simulink model "p_regler_bei_u_max"  (R2016b)
settings: Solver=VariableStepAuto  StartTime=0.0  StopTime=10.0  RelTol=1e-3
undefined symbols (not defined in the file or in its folder): K_P
libraries: simulink x1
settings Model: Creator=Fritz  LastModifiedBy=Fritz

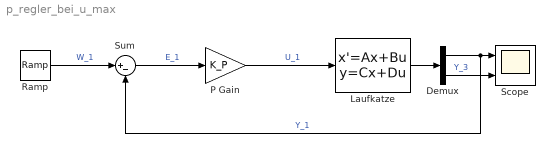
== system p_regler_bei_u_max ==
  Demux : Demux  Outputs=2
  Laufkatze : StateSpace  X0=0
  P Gain : Gain  Gain=K_P
  Ramp : simulink/Sources/Ramp  slope=0.1276  start=0  X0=0
  Scope : Scope  NumInputPorts=2
  Sum : Sum  Inputs=|+-
  wires:
  Demux/2 -> Scope/2  "Y_3"
  Sum/1 -> P Gain/1  "E_1"
  Demux/1 -> Sum/2, Scope/1  "Y_1"
  Ramp/1 -> Sum/1  "W_1"
  P Gain/1 -> Laufkatze/1  "U_1"
  Laufkatze/1 -> Demux/1
